simulink model "Decoder"  (R2020b)
settings: Solver=VariableStepAuto  StartTime=0.0  StopTime=10.0  RelTol=1e-3
libraries: uavmavlinklib x2
settings Model: Creator=macra  LastModifiedBy=macra

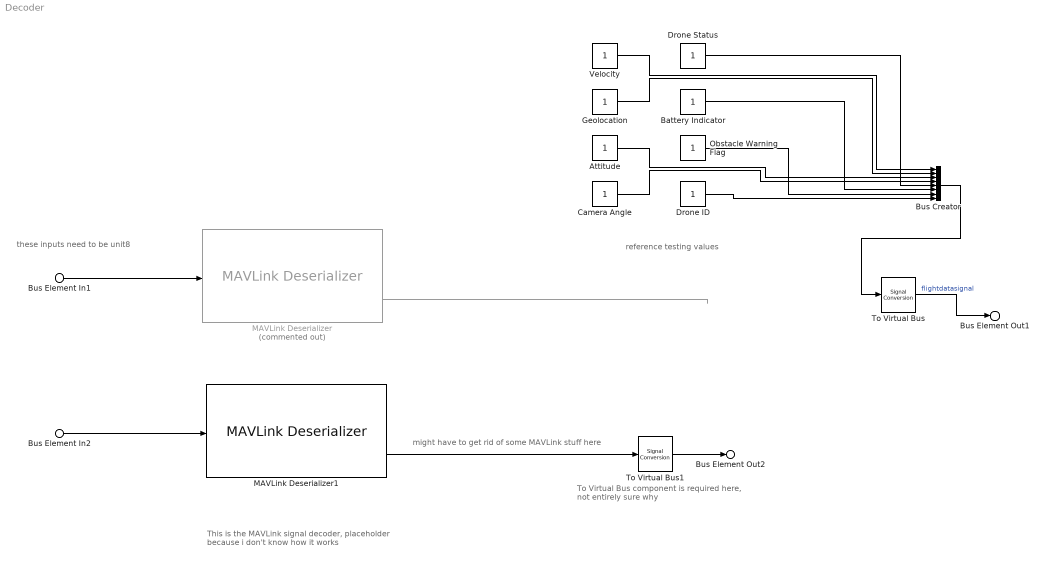
== system Decoder ==
  note: reference testing values
  note: To Virtual Bus component is required here,
      | not entirely sure why
  note: these inputs need to be
      | unit8
  note: might have to get rid of some MAVLink stuff here
  note: This is the MAVLink signal decoder, placeholder
      | because i don't know how it works
  Bus Element In1 : Inport  PortName=Decrypted Data From Drone
  Bus Element In2 : Inport  Port=2  PortName=Decrypted Video From Drone
  Attitude : Constant
  Battery Indicator : Constant
  Bus Creator : BusCreator  Inputs=8
  Camera Angle : Constant
  Drone ID : Constant
  Drone Status : Constant
  Geolocation : Constant
  MAVLink Deserializer : uavmavlinklib/MAVLink Deserializer  Commented=on  dialectSource=Select from standard MAVLink dialects  dialect=common.xml  dialectCustom=common.xml  version=2  messageType=HEARTBEAT  inputDataLength=off  SystemIDFilter=off  systemID=1  ComponentIDFilter=off  componentID=1  queueMsg=off  queueMsgSize=50  dropNum=off
      settings: SourceProductBaseCode=UV
  MAVLink Deserializer1 : uavmavlinklib/MAVLink Deserializer  dialectSource=Select from standard MAVLink dialects  dialect=common.xml  dialectCustom=common.xml  version=2  messageType=VIDEO_STREAM_INFORMATION  inputDataLength=off  SystemIDFilter=off  systemID=1  ComponentIDFilter=off  componentID=1  queueMsg=off  queueMsgSize=50  dropNum=off
      settings: SourceProductBaseCode=UV
  Obstacle Warning Flag : Constant
  To Virtual Bus : SignalConversion  ConversionOutput=Virtual bus  OverrideOpt=off
  To Virtual Bus1 : SignalConversion  ConversionOutput=Virtual bus  OverrideOpt=off
  Velocity : Constant
  Bus Element Out1 : Outport  PortName=Flight Data  Element=flightdatasignal
  Bus Element Out2 : Outport  Port=2  PortName=Camera Feed
  wires:
  Bus Element In1/1 -> MAVLink Deserializer/1
  Bus Element In2/1 -> MAVLink Deserializer1/1
  To Virtual Bus/1 -> Bus Element Out1/1  "flightdatasignal"
  MAVLink Deserializer/2 -> ?
  To Virtual Bus1/1 -> Bus Element Out2/1
  MAVLink Deserializer1/2 -> To Virtual Bus1/1
  Bus Creator/1 -> To Virtual Bus/1
  Velocity/1 -> Bus Creator/1
  Geolocation/1 -> Bus Creator/2
  Attitude/1 -> Bus Creator/3
  Camera Angle/1 -> Bus Creator/4
  Drone Status/1 -> Bus Creator/5
  Battery Indicator/1 -> Bus Creator/6
  Obstacle Warning Flag/1 -> Bus Creator/7
  Drone ID/1 -> Bus Creator/8
